simulink model "goldenDragonV2"  (R2017b)
settings: Solver=VariableStepAuto  StartTime=0.0  StopTime=4  RelTol=1e-3  EnableMultiTasking=on
PreLoadFcn:
  | goldenDragonData;
values from neighbouring files (symbols this model uses):
  b = 10000    [goldenDragonData.m]
  headMass = 150    [goldenDragonData.m]
  inputTs = 0.1    [goldenDragonData.m]
  k = 5000    [goldenDragonData.m]
  tailMass = 1    [goldenDragonData.m]
undefined symbols (not defined in the file or in its folder): X, Y, Z
libraries: fl_lib x33, sm_lib x9, nesl_utility x3, aerolibconvert2 x1
settings Model: Creator=scastro  LastModifiedBy=valakshe
settings DataIOCC: LimitDataPoints=on
settings OptimizationCC: LifeSpan=inf
settings DebuggingCC: AllowSymbolicDim=off  SFUnexpectedBacktrackingDiag=warning  SFNoUnconditionalDefaultTransitionDiag=warning  SFExecutionAtInitializationDiag=none
settings CodeAppCC: StateflowObjectComments=on
settings GRTTargetCC: TargetLangStandard=C89/C90 (ANSI)  GeneratePreprocessorConditionals=Disable all
settings ConfigComp: CovMetricSettings=dw  CovHtmlReporting=on  CovSaveCumulativeToWorkspaceVar=on  CovSaveSingleToWorkspaceVar=on  CovExternalEMLEnable=off  CovSFcnEnable=off
settings SimscapeCC: SimscapeNominalValues="[{\"value\":\"10\",\"unit\":\"V\"},{\"value\":\"1\",\"unit\":\"A\"},{\"value\":\"10\",\"unit\":\"N*m\"},{\"value\":\"10\",\"unit\":\"bar\"},{\"value\":\"100\",\"unit\":\"kJ/kg\"},{\"value\":\"1\",\"unit\":\"kW\"},{\"value\":\"300\",\"unit\":\"K\"},{\"value\":\"100\",\"unit\":\"cm^3/s\"},{\"value\":\"1\",\"unit\":\"kN\"},{\"value\":\"1\",\"unit\":\"g/cm^3\"},{\"value\":\"1\",\"unit\":\"l\"},{\"value\":\"1\",\"unit\":\"cm^2\"},{\"value\":\"60\",\"unit\":\"Hz\"}]"  SimscapeLogType=all  SimscapeLogDataHistory=10000
settings ConfigurationSet: Description=SimMechanics 2G
settings ExplorerConfigSet: InternalSimMechanicsExplorerSettings="<ExplorerConfiguration><canonicalview>default</canonicalview><AnimationSetting><BasePlaybackSpeed>1.0</BasePlaybackSpeed><PlaybackSpeedFactor>1.0</PlaybackSpeedFactor></AnimationSetting><TilePanel><TileInfo><Tiles Columns=\"1\" Count=\"1\" Rows=\"1\"><Column Weight=\"1\"/><Row Weight=\"1\"/><Tile Height=\"1\" Width=\"1\" X=\"0\" Y=\"0\"/></Tiles></TileInfo><SceneInfo><SceneViewer><BGColor><R>0.60000002384185791</R><G>0.60000002384185791</G><B>0.60000002384185791</B></BGColor><Camera><DoPerspective>off</DoPerspective><Position><X>39955.6705997624886</X><Y>-39954.0792290874306</Y><Z>39955.6205944664543</Z></Position><Center><X>0.248308761919401655</X><Y>1.34306191312877576</Y><Z>0.198303465895649539</Z></Center><Up><X>-0.408248290463863073</X><Y>0.408248290463863073</Y><Z>0.816496580927726145</Z></Up><ViewLimDist>1</ViewLimDist><YLim>1.18055898002874837</YLim><XLim>1.57024086390920559</XLim></Camera></SceneViewer></SceneInfo></TilePanel><MechEditorPanel><Cameras/><GfxPanelCameraMap/><VideoCreator><PlaybackSpeedRatio>1.0</PlaybackSpeedRatio><FrameRate>30</FrameRate><VideoFormat>Motion JPEG AVI</VideoFormat><FrameSize>auto</FrameSize></VideoCreator></MechEditorPanel></ExplorerConfiguration>"

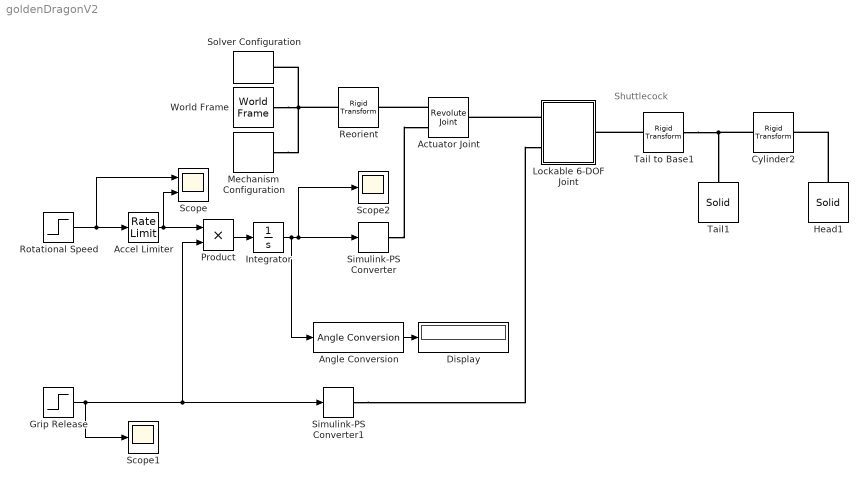
== system goldenDragonV2 ==
  note: Shuttlecock
  Accel Limiter : RateLimiter  RisingSlewLimit=5  FallingSlewLimit=-5  SampleTimeMode=inherited
  Actuator Joint : sm_lib/Joints/Revolute Joint  SenseConstraintForce=off  SenseConstraintForceX=off  SenseConstraintForceY=off  SenseConstraintForceZ=off  SenseConstraintTorque=off  SenseConstraintTorqueX=off  SenseConstraintTorqueY=off  SenseConstraintTorqueZ=off  SenseTotalForce=off  SenseTotalForceX=off  SenseTotalForceY=off  SenseTotalForceZ=off  SenseTotalTorque=off  SenseTotalTorqueX=off  SenseTotalTorqueY=off  SenseTotalTorqueZ=off  CompositeWrenchDir=FollowerOnBase  CompositeWrenchFrame=BaseFrame  EquilibriumPosition=0  EquilibriumPositionUnits=deg  SpringStiffness=0  SpringStiffnessUnits=N*m/deg  DampingCoefficient=0  DampingCoefficientUnits=N*m/(rad/s)  TorqueActuationMode=ComputedTorque  MotionActuationMode=InputMotion  SensePosition=off  SenseVelocity=off  SenseAcceleration=off  SenseTorqueForce=off  PositionTargetSpecify=off  PositionTargetPriority=High  PositionTargetValue=0  PositionTargetValueUnits=deg  VelocityTargetSpecify=off  VelocityTargetPriority=High  VelocityTargetValue=0  VelocityTargetValueUnits=deg/s
  Angle Conversion : aerolibconvert2/Angle Conversion  IU=rad  OU=rev
  Cylinder2 : sm_lib/Frames and Transforms/Rigid Transform  TranslationMethod=StandardAxis  TranslationStandardOffset=10  TranslationLengthUnit=cm  TranslationStandardAxis=+Z  TranslationCartesianOffset=[0 0 0]  TranslationROffset=0  TranslationROffsetUnits=m  TranslationZOffset=0  TranslationZOffsetUnits=m  TranslationThetaOffset=0  TranslationThetaOffsetUnits=deg  RotationMethod=StandardAxis  RotationAngleUnits=deg  RotationStandardAxis=+X  RotationAngle=90  RotationArbitraryAxis=[0 0 1]  FollAlignAxisA=+X  BaseAlignAxisA=+Y  FollAlignAxisB=+Y  BaseAlignAxisB=+Z  RotationSequenceAxes=FollowerAxes  RotationSequence=XYX  RotationSequenceAngles=[0 0 0]  RotationSequenceAnglesUnits=deg  RotationMatrix=[1 0 0; 0 1 0; 0 0 1]
  Display : Display
  Grip Release : Step  Time=2.6250  Before=1  After=0  SampleTime=0
  Head1 : sm_lib/Body Elements/Solid  InertiaType=CalculateFromGeometry  Mass=headMass  MassUnits=g  CenterOfMass=[0 0 0]  CenterOfMassUnits=m  MomentsOfInertia=[1 1 1]  MomentsOfInertiaUnits=kg*m^2  ProductsOfInertia=[1 1 1]  ProductsOfInertiaUnits=kg*m^2  DensityBased=off  Density=1000  DensityUnits=kg/m^3  DoExposeReferenceFrame=on  SerializedFrames=<Frames/>  GraphicType=FromGeometry  MarkerShape=Sphere  MarkerSize=10  GraphicVisPropType=SimpleVisualProperties  GraphicDiffuseColor=[1.0 0.0 0.0]  GraphicSpecularColor=[0.5 0.5 0.5 1.0]  GraphicAmbientColor=[0.15 0.15 0.15 1.0]  GraphicEmissiveColor=[0.0 0.0 0.0 1.0]  GraphicShininess=75  GraphicOpacity=1.0  GeometryShape=Sphere  RectangleSize=[1 1]  RectangleSizeUnits=m  BrickDimensions=[1 1 20]  BrickDimensionUnits=m  CylinderRadius=2.5  CylinderRadiusUnits=mm  CylinderLength=20  CylinderLengthUnits=cm  SphereRadius=2  SphereRadiusUnits=cm  EllipsoidRadii=[1 1 1]  EllipsoidRadiiUnits=m  ExtrusionCrossSection=[1 1; -1 1; -1 -1; 1 -1]  ExtrusionCrossSectionUnits=m  ExtrusionLength=1  ExtrusionLengthUnits=m  PolygonNumSides=3  PolygonOuterRadius=1  PolygonOuterRadiusUnits=m  ExtGeomFileType=STEP  ExtGeomFileUnits=m  RevolutionCrossSection=[1 1; 1 -1; 2 -1; 2 1]  RevolutionCrossSectionUnits=m  RevolutionExtent=Full  RevolutionAngle=180  RevolutionAngleUnits=deg
  Integrator : Integrator
  Lockable 6-DOF Joint : Subsystem
  Mechanism Configuration : sm_lib/Utilities/Mechanism Configuration  UniformGravity=Constant  GravityVector=[0 0 -9.80665]  GravityUnits=m/s^2  LinearizationDelta=0.001
  Product : Product
  Reorient : sm_lib/Frames and Transforms/Rigid Transform  TranslationMethod=None  TranslationStandardOffset=0  TranslationLengthUnit=m  TranslationStandardAxis=+Z  TranslationCartesianOffset=[0 0 0]  TranslationROffset=0  TranslationROffsetUnits=m  TranslationZOffset=0  TranslationZOffsetUnits=m  TranslationThetaOffset=0  TranslationThetaOffsetUnits=deg  RotationMethod=StandardAxis  RotationAngleUnits=deg  RotationStandardAxis=+Y  RotationAngle=90  RotationArbitraryAxis=[0 0 1]  FollAlignAxisA=+X  BaseAlignAxisA=+Y  FollAlignAxisB=+Y  BaseAlignAxisB=+Z  RotationSequenceAxes=FollowerAxes  RotationSequence=XYX  RotationSequenceAngles=[0 0 0]  RotationSequenceAnglesUnits=deg  RotationMatrix=[1 0 0; 0 1 0; 0 0 1]
  Rotational Speed : Step  Time=0  After=30  SampleTime=inputTs
  Scope : Scope  NumInputPorts=2
  Scope1 : Scope
  Scope2 : Scope
  Simulink-PS Converter : nesl_utility/Simulink-PS Converter  PhysicalDomain=network_engine_domain  SubClassName=ps_input  LeftPortType=input  RightPortType=output  PseudoPeriodic=off  Frequencies=[]  NoiseDistribution=none  NoiseParameters=[]  Unit=rad  AffineConversion=off  FilteringAndDerivatives=filter  SimscapeFilterOrder=2  InputFilterTimeConstant=inputFiltConstant  UdotUserProvided=1
  Simulink-PS Converter1 : nesl_utility/Simulink-PS Converter  PhysicalDomain=network_engine_domain  SubClassName=ps_input  LeftPortType=input  RightPortType=output  PseudoPeriodic=off  Frequencies=[]  NoiseDistribution=none  NoiseParameters=[]  Unit=1  AffineConversion=off  FilteringAndDerivatives=provide  SimscapeFilterOrder=2  InputFilterTimeConstant=inputFiltConstant  UdotUserProvided=0
  Solver Configuration : nesl_utility/Solver Configuration  PhysicalDomain=network_engine_domain  SubClassName=solver  LeftPortType=input  RightPortType=generic  Accelerate=off  Tones=[]  Harmonics=[]  SimulateNoise=off  Profile=off  UseLocalSampling=off  EnableSwitchedLinearOptims=on  FrequencyDomain=off  UseCCode=off  RelTol=0.001  AbsTol=1e-06  MinStep=1e-09  ToWorkspace=off  RevertToSquareIcSolve=off  NumHomotopyIterations=100  PhasorMode=off  PhasorModeNumHarmonics=1  DoDC=off  ResidualTolerance=1e-09  UseLocalSolver=off  LocalSolverChoice=NE_BACKWARD_EULER_ADVANCER  LocalSolverSampleTime=0.001  DoFixedCost=off  MaxNonlinIter=3  MaxModeIter=2  LinearAlgebra=Sparse  DelaysMemoryBudget=1024  AutomaticFiltering=on  FilteringTimeConstant=0.001
  Tail to Base1 : sm_lib/Frames and Transforms/Rigid Transform  TranslationMethod=StandardAxis  TranslationStandardOffset=10  TranslationLengthUnit=cm  TranslationStandardAxis=-Z  TranslationCartesianOffset=[0 0 0]  TranslationROffset=0  TranslationROffsetUnits=m  TranslationZOffset=0  TranslationZOffsetUnits=m  TranslationThetaOffset=0  TranslationThetaOffsetUnits=deg  RotationMethod=StandardAxis  RotationAngleUnits=deg  RotationStandardAxis=+X  RotationAngle=90  RotationArbitraryAxis=[0 0 1]  FollAlignAxisA=+X  BaseAlignAxisA=+Y  FollAlignAxisB=+Y  BaseAlignAxisB=+Z  RotationSequenceAxes=FollowerAxes  RotationSequence=XYX  RotationSequenceAngles=[0 0 0]  RotationSequenceAnglesUnits=deg  RotationMatrix=[1 0 0; 0 1 0; 0 0 1]
  Tail1 : sm_lib/Body Elements/Solid  InertiaType=CalculateFromGeometry  Mass=tailMass  MassUnits=g  CenterOfMass=[0 0 0]  CenterOfMassUnits=m  MomentsOfInertia=[1 1 1]  MomentsOfInertiaUnits=kg*m^2  ProductsOfInertia=[1 1 1]  ProductsOfInertiaUnits=kg*m^2  DensityBased=off  Density=1000  DensityUnits=kg/m^3  DoExposeReferenceFrame=on  SerializedFrames=<Frames/>  GraphicType=FromGeometry  MarkerShape=Sphere  MarkerSize=10  GraphicVisPropType=SimpleVisualProperties  GraphicDiffuseColor=[1.0 0.0 0.0]  GraphicSpecularColor=[0.5 0.5 0.5 1.0]  GraphicAmbientColor=[0.15 0.15 0.15 1.0]  GraphicEmissiveColor=[0.0 0.0 0.0 1.0]  GraphicShininess=75  GraphicOpacity=1.0  GeometryShape=Cylinder  RectangleSize=[1 1]  RectangleSizeUnits=m  BrickDimensions=[1 1 20]  BrickDimensionUnits=m  CylinderRadius=2.5  CylinderRadiusUnits=mm  CylinderLength=20  CylinderLengthUnits=cm  SphereRadius=1  SphereRadiusUnits=m  EllipsoidRadii=[1 1 1]  EllipsoidRadiiUnits=m  ExtrusionCrossSection=[1 1; -1 1; -1 -1; 1 -1]  ExtrusionCrossSectionUnits=m  ExtrusionLength=1  ExtrusionLengthUnits=m  PolygonNumSides=3  PolygonOuterRadius=1  PolygonOuterRadiusUnits=m  ExtGeomFileType=STEP  ExtGeomFileUnits=m  RevolutionCrossSection=[1 1; 1 -1; 2 -1; 2 1]  RevolutionCrossSectionUnits=m  RevolutionExtent=Full  RevolutionAngle=180  RevolutionAngleUnits=deg
  World Frame : sm_lib/Frames and Transforms/World Frame
  wires:
  Grip Release/1 -> Simulink-PS Converter1/1, Product/2, Scope1/1
  Rotational Speed/1 -> Scope/1, Accel Limiter/1
  Accel Limiter/1 -> Scope/2, Product/1
  Integrator/1 -> Angle Conversion/1, Simulink-PS Converter/1, Scope2/1
  Product/1 -> Integrator/1
  Angle Conversion/1 -> Display/1
  connections:
  Mechanism Configuration/RConn1 -- Reorient/LConn1 -- Solver Configuration/RConn1 -- World Frame/RConn1
  Actuator Joint/LConn1 -- Reorient/RConn1
  Tail to Base1/RConn1 -- Lockable 6-DOF Joint/RConn1
  Cylinder2/LConn1 -- Tail1/RConn1 -- Tail to Base1/LConn1
  Head1/RConn1 -- Cylinder2/RConn1
  Simulink-PS Converter1/RConn1 -- Lockable 6-DOF Joint/LConn2
  Lockable 6-DOF Joint/LConn1 -- Actuator Joint/RConn1
  Simulink-PS Converter/RConn1 -- Actuator Joint/LConn2

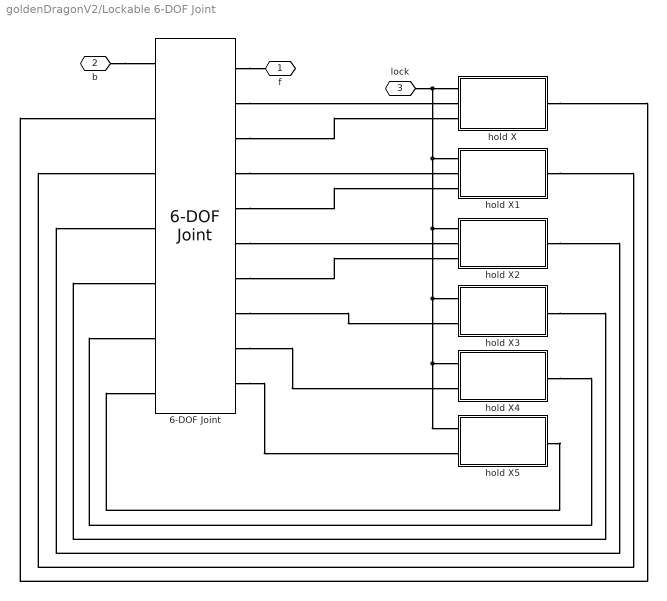
== system goldenDragonV2/Lockable 6-DOF Joint ==
  6-DOF Joint : sm_lib/Joints/6-DOF Joint  SenseConstraintForce=off  SenseConstraintForceX=off  SenseConstraintForceY=off  SenseConstraintForceZ=off  SenseConstraintTorque=off  SenseConstraintTorqueX=off  SenseConstraintTorqueY=off  SenseConstraintTorqueZ=off  SenseTotalForce=off  SenseTotalForceX=off  SenseTotalForceY=off  SenseTotalForceZ=off  SenseTotalTorque=off  SenseTotalTorqueX=off  SenseTotalTorqueY=off  SenseTotalTorqueZ=off  CompositeWrenchDir=FollowerOnBase  CompositeWrenchFrame=BaseFrame  PxEquilibriumPosition=0  PxEquilibriumPositionUnits=m  PxSpringStiffness=0  PxSpringStiffnessUnits=N/m  PxDampingCoefficient=prisDamping  PxDampingCoefficientUnits=N/(m/s)  PxTorqueActuationMode=InputTorque  PxMotionActuationMode=ComputedMotion  PxSensePosition=on  PxSenseVelocity=on  PxSenseAcceleration=off  PxSenseTorqueForce=off  PxPositionTargetSpecify=off  PxPositionTargetPriority=High  PxPositionTargetValue=0  PxPositionTargetValueUnits=m  PxVelocityTargetSpecify=off  PxVelocityTargetPriority=High  PxVelocityTargetValue=0  PxVelocityTargetValueUnits=m/s  PyEquilibriumPosition=0  PyEquilibriumPositionUnits=m  PySpringStiffness=0  PySpringStiffnessUnits=N/m  PyDampingCoefficient=prisDamping  PyDampingCoefficientUnits=N/(m/s)  PyTorqueActuationMode=InputTorque  PyMotionActuationMode=ComputedMotion  PySensePosition=on  PySenseVelocity=on  PySenseAcceleration=off  PySenseTorqueForce=off  PyPositionTargetSpecify=off  PyPositionTargetPriority=High  PyPositionTargetValue=0  PyPositionTargetValueUnits=m  PyVelocityTargetSpecify=off  PyVelocityTargetPriority=High  PyVelocityTargetValue=0  PyVelocityTargetValueUnits=m/s  PzEquilibriumPosition=0  PzEquilibriumPositionUnits=m  PzSpringStiffness=0  PzSpringStiffnessUnits=N/m  PzDampingCoefficient=prisDamping  PzDampingCoefficientUnits=N/(m/s)  PzTorqueActuationMode=InputTorque  PzMotionActuationMode=ComputedMotion  PzSensePosition=on  PzSenseVelocity=on  PzSenseAcceleration=off  PzSenseTorqueForce=off  PzPositionTargetSpecify=off  PzPositionTargetPriority=High  PzPositionTargetValue=0  PzPositionTargetValueUnits=m  PzVelocityTargetSpecify=off  PzVelocityTargetPriority=High  PzVelocityTargetValue=0  PzVelocityTargetValueUnits=m/s  SphDefPosRotationMethod=None  SphDefPosRotationAngleUnits=deg  SphDefPosRotationStandardAxis=+Z  SphDefPosRotationAngle=0.0  SphDefPosRotationArbitraryAxis=[0 0 1]  SphDefPosFollAlignAxisA=+X  SphDefPosBaseAlignAxisA=+Y  SphDefPosFollAlignAxisB=+Y  SphDefPosBaseAlignAxisB=+Z  SphDefPosRotationSequenceAxes=FollowerAxes  SphDefPosRotationSequence=XYX  SphDefPosRotationSequenceAngles=[0 0 0]  SphDefPosRotationSequenceAnglesUnits=deg  SphDefPosRotationMatrix=[1 0 0; 0 1 0; 0 0 1]  SphEqPosRotationMethod=None  SphEqPosRotationAngleUnits=deg  SphEqPosRotationStandardAxis=+Z  SphEqPosRotationAngle=0.0  SphEqPosRotationArbitraryAxis=[0 0 1]  SphEqPosFollAlignAxisA=+X  SphEqPosBaseAlignAxisA=+Y  SphEqPosFollAlignAxisB=+Y  SphEqPosBaseAlignAxisB=+Z  SphEqPosRotationSequenceAxes=FollowerAxes  SphEqPosRotationSequence=XYX  SphEqPosRotationSequenceAngles=[0 0 0]  SphEqPosRotationSequenceAnglesUnits=deg  SphEqPosRotationMatrix=[1 0 0; 0 1 0; 0 0 1]  SphSpringStiffness=0  SphSpringStiffnessUnits=N*m/deg  SphDampingCoefficient=jointDamping  SphDampingCoefficientUnits=N*m/(rad/s)  SphActuateTorqueX=on  SphActuateTorqueY=on  SphActuateTorqueZ=on  SphActuateTorque=off  SphTorqueActuationMode=InputTorque  SphMotionActuationMode=ComputedMotion  SphActuationFrame=BaseFrame  SphSensePosition=off  SphSenseVelocityX=on  SphSenseVelocityY=on  SphSenseVelocityZ=on  SphSenseVelocity=off  SphSenseAccelerationX=off  SphSenseAccelerationY=off  SphSenseAccelerationZ=off  SphSenseAcceleration=off  SphSenseTorqueX=off  SphSenseTorqueY=off  SphSenseTorqueZ=off  SphSenseTorqueForce=off  SphSensingFrame=FollowerFrame  SphPositionTargetRotationMethod=None  SphPositionTargetRotationAngleUnits=deg  SphPositionTargetRotationStandardAxis=+Z  SphPositionTargetRotationAngle=0.0  SphPositionTargetRotationArbitraryAxis=[0 0 1]  SphPositionTargetFollAlignAxisA=+X  SphPositionTargetBaseAlignAxisA=+Y  SphPositionTargetFollAlignAxisB=+Y  SphPositionTargetBaseAlignAxisB=+Z  SphPositionTargetRotationSequenceAxes=FollowerAxes  SphPositionTargetRotationSequence=XYX  SphPositionTargetRotationSequenceAngles=[0 0 0]  SphPositionTargetRotationSequenceAnglesUnits=deg  SphPositionTargetRotationMatrix=[1 0 0; 0 1 0; 0 0 1]  SphPositionTargetSpecify=off  SphPositionTargetPriority=High  SphVelocityTargetValue=[0 0 0]  SphVelocityTargetValueUnits=deg/s  SphVelocityTargetSpecify=off  SphVelocityTargetPriority=High  SphVelocityTargetInFollowerFrame=on
  hold X : Subsystem
  hold X1 : Subsystem
  hold X2 : Subsystem
  hold X3 : Subsystem
  hold X4 : Subsystem
  hold X5 : Subsystem
  f : PMIOPort  Port=1  Side=Right
  b : PMIOPort  Port=2  Side=Left
  lock : PMIOPort  Port=3  Side=Left
  connections:
  lock/RConn1 -- hold X/LConn1 -- hold X5/LConn1 -- hold X4/LConn1 -- hold X3/LConn1 -- hold X2/LConn1 -- hold X1/LConn1
  6-DOF Joint/RConn9 -- hold X4/LConn2
  6-DOF Joint/RConn8 -- hold X3/LConn2
  hold X/RConn1 -- 6-DOF Joint/LConn2
  b/RConn1 -- 6-DOF Joint/LConn1
  6-DOF Joint/RConn10 -- hold X5/LConn2
  hold X1/RConn1 -- 6-DOF Joint/LConn3
  6-DOF Joint/RConn2 -- hold X/LConn2
  6-DOF Joint/RConn6 -- hold X2/LConn2
  6-DOF Joint/RConn3 -- hold X/LConn3
  6-DOF Joint/RConn7 -- hold X2/LConn3
  hold X3/RConn1 -- 6-DOF Joint/LConn5
  6-DOF Joint/RConn4 -- hold X1/LConn2
  6-DOF Joint/RConn5 -- hold X1/LConn3
  6-DOF Joint/RConn1 -- f/RConn1
  hold X4/RConn1 -- 6-DOF Joint/LConn6
  hold X2/RConn1 -- 6-DOF Joint/LConn4
  hold X5/RConn1 -- 6-DOF Joint/LConn7

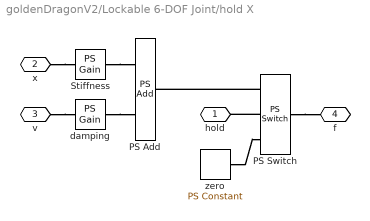
== system goldenDragonV2/Lockable 6-DOF Joint/hold X ==
  PS Add : fl_lib/Physical Signals/Functions/PS Add
  PS Switch : fl_lib/Physical Signals/Nonlinear Operators/PS Switch  Threshold=0.5
      settings: SourceProductName=Simscape  SourceProductBaseCode=SS
  Stiffness : fl_lib/Physical Signals/Functions/PS Gain  gain=-k
  damping : fl_lib/Physical Signals/Functions/PS Gain  gain=-b
  zero : fl_lib/Physical Signals/Sources/PS Constant  constant=0
  hold : PMIOPort  Port=1  Side=Left
  x : PMIOPort  Port=2  Side=Left
  v : PMIOPort  Port=3  Side=Left
  f : PMIOPort  Port=4  Side=Right
  connections:
  PS Switch/LConn1 -- PS Add/RConn1
  v/RConn1 -- damping/LConn1
  x/RConn1 -- Stiffness/LConn1
  zero/RConn1 -- PS Switch/LConn3
  Stiffness/RConn1 -- PS Add/LConn1
  damping/RConn1 -- PS Add/LConn2
  PS Switch/RConn1 -- f/RConn1
  PS Switch/LConn2 -- hold/RConn1

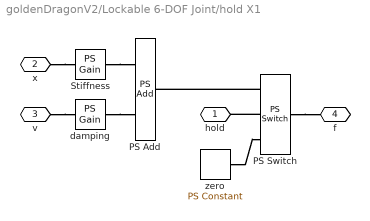
== system goldenDragonV2/Lockable 6-DOF Joint/hold X1 ==
  PS Add : fl_lib/Physical Signals/Functions/PS Add
  PS Switch : fl_lib/Physical Signals/Nonlinear Operators/PS Switch  Threshold=0.5
      settings: SourceProductName=Simscape  SourceProductBaseCode=SS
  Stiffness : fl_lib/Physical Signals/Functions/PS Gain  gain=-k
  damping : fl_lib/Physical Signals/Functions/PS Gain  gain=-b
  zero : fl_lib/Physical Signals/Sources/PS Constant  constant=0
  hold : PMIOPort  Port=1  Side=Left
  x : PMIOPort  Port=2  Side=Left
  v : PMIOPort  Port=3  Side=Left
  f : PMIOPort  Port=4  Side=Right
  connections:
  PS Switch/LConn2 -- hold/RConn1
  PS Switch/RConn1 -- f/RConn1
  damping/RConn1 -- PS Add/LConn2
  Stiffness/RConn1 -- PS Add/LConn1
  zero/RConn1 -- PS Switch/LConn3
  x/RConn1 -- Stiffness/LConn1
  v/RConn1 -- damping/LConn1
  PS Switch/LConn1 -- PS Add/RConn1

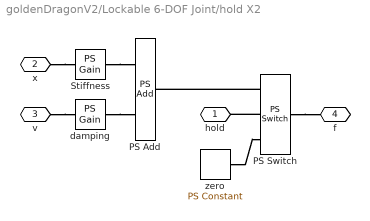
== system goldenDragonV2/Lockable 6-DOF Joint/hold X2 ==
  PS Add : fl_lib/Physical Signals/Functions/PS Add
  PS Switch : fl_lib/Physical Signals/Nonlinear Operators/PS Switch  Threshold=0.5
      settings: SourceProductName=Simscape  SourceProductBaseCode=SS
  Stiffness : fl_lib/Physical Signals/Functions/PS Gain  gain=-k
  damping : fl_lib/Physical Signals/Functions/PS Gain  gain=-b
  zero : fl_lib/Physical Signals/Sources/PS Constant  constant=0
  hold : PMIOPort  Port=1  Side=Left
  x : PMIOPort  Port=2  Side=Left
  v : PMIOPort  Port=3  Side=Left
  f : PMIOPort  Port=4  Side=Right
  connections:
  PS Switch/LConn1 -- PS Add/RConn1
  v/RConn1 -- damping/LConn1
  x/RConn1 -- Stiffness/LConn1
  zero/RConn1 -- PS Switch/LConn3
  Stiffness/RConn1 -- PS Add/LConn1
  damping/RConn1 -- PS Add/LConn2
  PS Switch/RConn1 -- f/RConn1
  PS Switch/LConn2 -- hold/RConn1

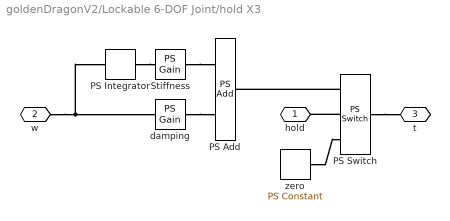
== system goldenDragonV2/Lockable 6-DOF Joint/hold X3 ==
  PS Add : fl_lib/Physical Signals/Functions/PS Add
  PS Integrator : fl_lib/Physical Signals/Linear Operators/PS Integrator  x0=0
      settings: SourceProductName=Simscape  SourceProductBaseCode=SS
  PS Switch : fl_lib/Physical Signals/Nonlinear Operators/PS Switch  Threshold=0.5
      settings: SourceProductName=Simscape  SourceProductBaseCode=SS
  Stiffness : fl_lib/Physical Signals/Functions/PS Gain  gain=-k
  damping : fl_lib/Physical Signals/Functions/PS Gain  gain=-b
  zero : fl_lib/Physical Signals/Sources/PS Constant  constant=0
  hold : PMIOPort  Port=1  Side=Left
  w : PMIOPort  Port=2  Side=Left
  t : PMIOPort  Port=3  Side=Right
  connections:
  PS Switch/LConn2 -- hold/RConn1
  PS Switch/RConn1 -- t/RConn1
  damping/RConn1 -- PS Add/LConn2
  Stiffness/RConn1 -- PS Add/LConn1
  zero/RConn1 -- PS Switch/LConn3
  w/RConn1 -- PS Integrator/LConn1 -- damping/LConn1
  PS Switch/LConn1 -- PS Add/RConn1
  PS Integrator/RConn1 -- Stiffness/LConn1

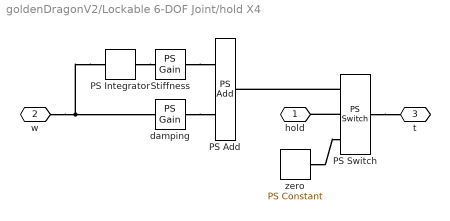
== system goldenDragonV2/Lockable 6-DOF Joint/hold X4 ==
  PS Add : fl_lib/Physical Signals/Functions/PS Add
  PS Integrator : fl_lib/Physical Signals/Linear Operators/PS Integrator  x0=0
      settings: SourceProductName=Simscape  SourceProductBaseCode=SS
  PS Switch : fl_lib/Physical Signals/Nonlinear Operators/PS Switch  Threshold=0.5
      settings: SourceProductName=Simscape  SourceProductBaseCode=SS
  Stiffness : fl_lib/Physical Signals/Functions/PS Gain  gain=-k
  damping : fl_lib/Physical Signals/Functions/PS Gain  gain=-b
  zero : fl_lib/Physical Signals/Sources/PS Constant  constant=0
  hold : PMIOPort  Port=1  Side=Left
  w : PMIOPort  Port=2  Side=Left
  t : PMIOPort  Port=3  Side=Right
  connections:
  PS Integrator/RConn1 -- Stiffness/LConn1
  PS Switch/LConn1 -- PS Add/RConn1
  PS Integrator/LConn1 -- w/RConn1 -- damping/LConn1
  zero/RConn1 -- PS Switch/LConn3
  Stiffness/RConn1 -- PS Add/LConn1
  damping/RConn1 -- PS Add/LConn2
  PS Switch/RConn1 -- t/RConn1
  PS Switch/LConn2 -- hold/RConn1

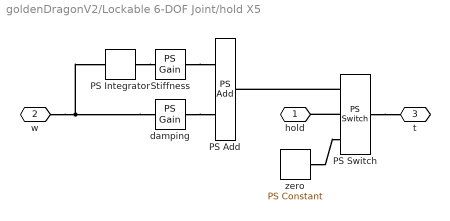
== system goldenDragonV2/Lockable 6-DOF Joint/hold X5 ==
  PS Add : fl_lib/Physical Signals/Functions/PS Add
  PS Integrator : fl_lib/Physical Signals/Linear Operators/PS Integrator  x0=0
      settings: SourceProductName=Simscape  SourceProductBaseCode=SS
  PS Switch : fl_lib/Physical Signals/Nonlinear Operators/PS Switch  Threshold=0.5
      settings: SourceProductName=Simscape  SourceProductBaseCode=SS
  Stiffness : fl_lib/Physical Signals/Functions/PS Gain  gain=-k
  damping : fl_lib/Physical Signals/Functions/PS Gain  gain=-b
  zero : fl_lib/Physical Signals/Sources/PS Constant  constant=0
  hold : PMIOPort  Port=1  Side=Left
  w : PMIOPort  Port=2  Side=Left
  t : PMIOPort  Port=3  Side=Right
  connections:
  PS Switch/LConn2 -- hold/RConn1
  PS Switch/RConn1 -- t/RConn1
  damping/RConn1 -- PS Add/LConn2
  Stiffness/RConn1 -- PS Add/LConn1
  zero/RConn1 -- PS Switch/LConn3
  damping/LConn1 -- w/RConn1 -- PS Integrator/LConn1
  PS Switch/LConn1 -- PS Add/RConn1
  PS Integrator/RConn1 -- Stiffness/LConn1
